simulink model "BiCycleModel"  (R2019a)
settings: Solver=ode3  StartTime=0.0  StopTime=inf  FixedStep=0.01  RelTol=1e-3
libraries: robotlib x1
settings Model: Creator=ivory  LastModifiedBy=ivory

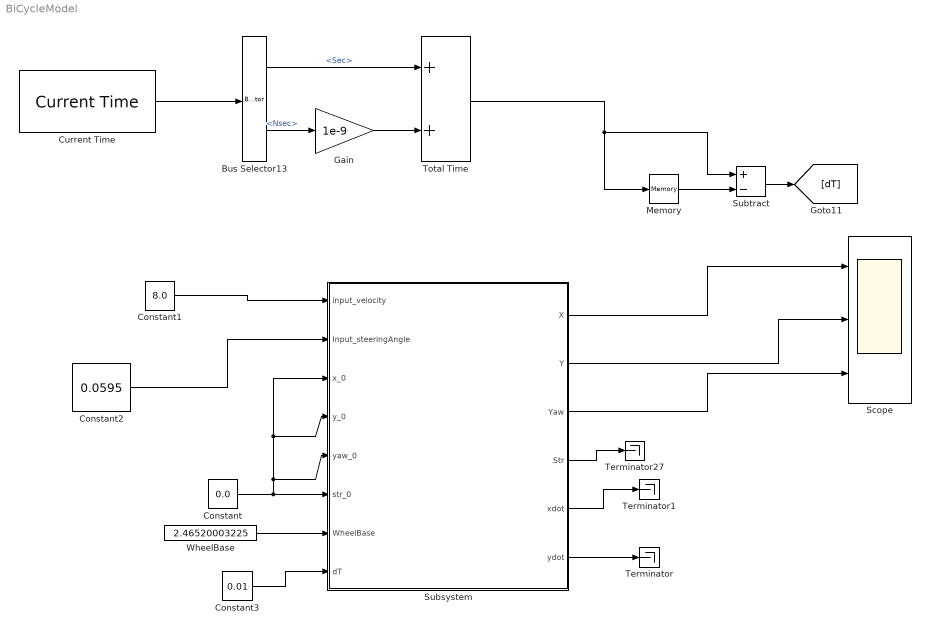
== system BiCycleModel ==
  Bus Selector13 : BusSelector  OutputSignals=Sec,Nsec
  Constant : Constant  Value=0.0
  Constant1 : Constant  Value=8.0
  Constant2 : Constant  Value=0.0595
  Constant3 : Constant  Value=0.01
  Current Time : robotlib/Current Time  OutputFormat=bus  SampleTime=-1  ModelName=BiCycleModel
      settings: SourceProductName=Robotics System Toolbox  SourceProductBaseCode=RO
  Gain : Gain  Gain=1e-9
  Memory : Memory
  Scope : Scope  NumInputPorts=3
  Subsystem : Subsystem
  Subtract : Sum  Inputs=+-
  Terminator : Terminator
  Terminator1 : Terminator
  Terminator27 : Terminator
  Total Time : Sum
  WheelBase : Constant  Value=2.46520003225
  wires:
  Constant/1 -> Subsystem/4(y_0), Subsystem/3(x_0), Subsystem/5(yaw_0), Subsystem/6(str_0)
  WheelBase/1 -> Subsystem/7(WheelBase)
  Subsystem/4(Str) -> Terminator27/1
  Current Time/1 -> Bus Selector13/1
  Gain/1 -> Total Time/2
  Bus Selector13/1 -> Total Time/1  "<Sec>"
  Bus Selector13/2 -> Gain/1  "<Nsec>"
  Memory/1 -> Subtract/2
  Total Time/1 -> Subtract/1, Memory/1
  Subtract/1 -> [dT]
  Constant1/1 -> Subsystem/1(input_velocity)
  Constant2/1 -> Subsystem/2(Input_steeringAngle)
  Subsystem/1(X) -> Scope/1
  Subsystem/2(Y) -> Scope/2
  Subsystem/3(Yaw) -> Scope/3
  Subsystem/5(xdot) -> Terminator1/1
  Subsystem/6(ydot) -> Terminator/1
  Constant3/1 -> Subsystem/8(dT)

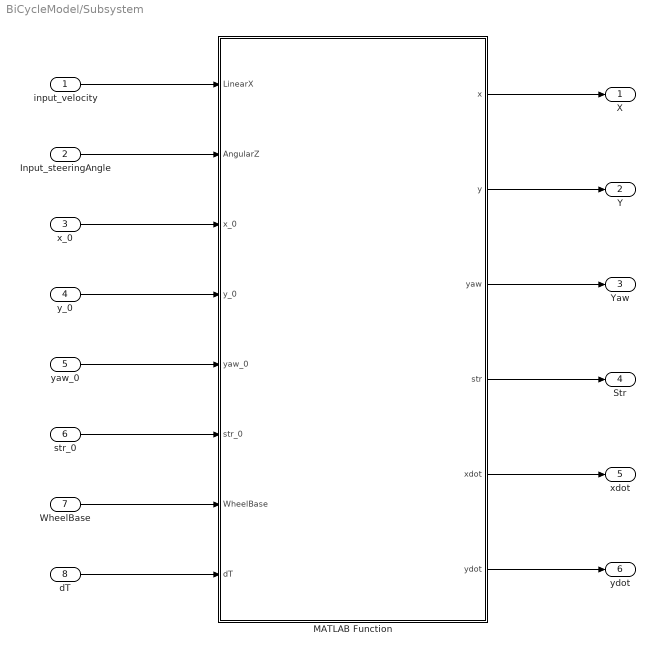
== system BiCycleModel/Subsystem ==
  input_velocity : Inport
  Input_steeringAngle : Inport  Port=2
  x_0 : Inport  Port=3
  y_0 : Inport  Port=4
  yaw_0 : Inport  Port=5
  str_0 : Inport  Port=6
  WheelBase : Inport  Port=7
  dT : Inport  Port=8
  MATLAB Function : MATLAB Function  TreatAsAtomicUnit=on
  X : Outport
  Y : Outport  Port=2
  Yaw : Outport  Port=3
  Str : Outport  Port=4
  xdot : Outport  Port=5
  ydot : Outport  Port=6
  wires:
  input_velocity/1 -> MATLAB Function/1(LinearX)
  Input_steeringAngle/1 -> MATLAB Function/2(AngularZ)
  x_0/1 -> MATLAB Function/3(x_0)
  y_0/1 -> MATLAB Function/4(y_0)
  yaw_0/1 -> MATLAB Function/5(yaw_0)
  str_0/1 -> MATLAB Function/6(str_0)
  WheelBase/1 -> MATLAB Function/7(WheelBase)
  MATLAB Function/1(x) -> X/1
  MATLAB Function/2(y) -> Y/1
  MATLAB Function/3(yaw) -> Yaw/1
  MATLAB Function/4(str) -> Str/1
  MATLAB Function/5(xdot) -> xdot/1
  MATLAB Function/6(ydot) -> ydot/1
  dT/1 -> MATLAB Function/8(dT)

== matlab function BiCycleModel/Subsystem/MATLAB Function ==
  data: x output; y output; LinearX input; AngularZ input; x_0 input; y_0 input; yaw_0 input; yaw output; str_0 input; WheelBase input; str output; xdot output; ydot output; dT input
function [x, y, yaw, str, xdot, ydot] = BicycleModel(LinearX,  AngularZ, x_0, y_0, yaw_0, str_0, WheelBase, dT)
    

    persistent x_old y_old yaw_old str_old

    if isempty(x_old)
        x_old = x_0;
    end
    
    if isempty(y_old)
        y_old = y_0;
    end
    
    if isempty(yaw_old)
        yaw_old = yaw_0;
    end
    
    if isempty(str_old)
        str_old = str_0;
    end
    
    
    % Rate of change of tire angle
    u2 = (AngularZ - str_old)/dT;
    
    xdot = LinearX*cos(str_old)*cos(yaw_old);
    ydot = LinearX*cos(str_old)*sin(yaw_old);
    x = x_old + dT*xdot;
    y = y_old + dT*ydot;
    
    str = str_old + dT*u2;
    
    if(str >0.5236)
        str = 0.5236;
    end
    
    if(str < - 0.5236)
        str = -0.5236;
    end
    
    yaw = yaw_old + dT*LinearX*(1/WheelBase)*sin(str_old);
    
    while(yaw < 0)
        yaw = yaw + 2*pi;
    end
    
    while(yaw > 2*pi)
        yaw = yaw - 2*pi;
    end
    
    x_old = x;
    y_old = y;
    str_old = str;
    yaw_old = yaw;
  
end
